simulink subsystem "High_Level_Controller"  (R2023a)
settings: Solver=VariableStepAuto  StartTime=0.0  StopTime=10.0  RelTol=1e-3
values from neighbouring files (symbols this model uses):
  k_d = 1    [constants.m]
  k_i = 1    [constants.m]
  k_p = 1    [constants.m]
settings Model: Creator=ycheb  LastModifiedBy=ycheb

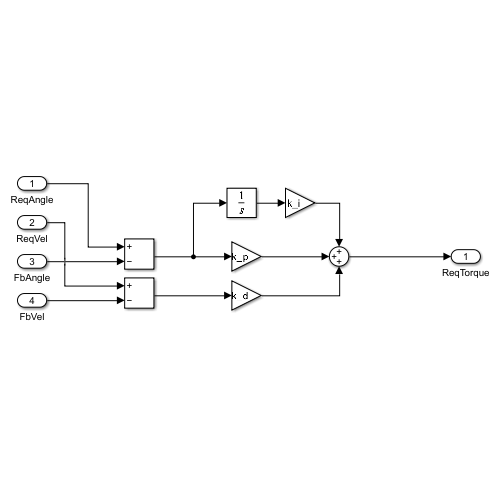
[thumbnail: Simulink's stored preview of the top-level diagram]
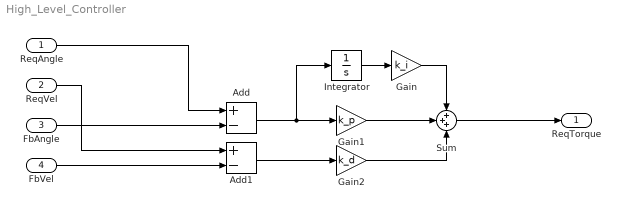
== system High_Level_Controller ==
  ReqAngle : Inport
  ReqVel : Inport  Port=2
  FbAngle : Inport  Port=3
  FbVel : Inport  Port=4
  Add : Sum  Inputs=+-
  Add1 : Sum  Inputs=+-
  Gain : Gain  Gain=k_i
  Gain1 : Gain  Gain=k_p
  Gain2 : Gain  Gain=k_d
  Integrator : Integrator
  Sum : Sum  Inputs=+++
  ReqTorque : Outport
  wires:
  Integrator/1 -> Gain/1
  Add/1 -> Integrator/1, Gain1/1
  Gain/1 -> Sum/1
  Gain1/1 -> Sum/2
  ReqAngle/1 -> Add/1
  ReqVel/1 -> Add1/1
  Add1/1 -> Gain2/1
  Sum/1 -> ReqTorque/1
  Gain2/1 -> Sum/3
  FbVel/1 -> Add1/2
  FbAngle/1 -> Add/2
